simulink model "PedalCmd"  (R2016a)
settings: Solver=FixedStepDiscrete  StartTime=0.0  StopTime=2  FixedStep=0.1  RelTol=1e-3
PostLoadFcn:
  | CruiseControl_dd;
undefined symbols (not defined in the file): PedalCmdY, SpeedDelX
settings Model: Creator=The MathWorks Inc.  LastModifiedBy=colosky
settings DataIOCC: LimitDataPoints=on  SaveFormat=Array  SaveOutput=off  SaveTime=off
settings OptimizationCC: ConditionallyExecuteInputs=off  DefaultParameterBehavior=Inlined  InlineInvariantSignals=on  ExpressionDepthLimit=2147483647  InitFltsAndDblsToZero=on  NoFixptDivByZeroProtection=on  OptimizeModelRefInitCode=on
settings DebuggingCC: SaveWithParameterizedLinksMsg=none  UnderspecifiedInitializationDetection=Classic  MergeDetectMultiDrivingBlocksExec=none  SolverPrmCheckMsg=warning  FcnCallInpInsideContextMsg=UseLocalSettings  AllowSymbolicDim=off  StateNameClashWarn=warning  StrictBusMsg=ErrorOnBusTreatedAsVector
settings HardwareCC: ProdBitPerPointer=32  ProdLargestAtomicFloat=None  ProdIntDivRoundTo=Undefined  ProdEndianess=Unspecified  ProdWordSize=32  ProdHWDeviceType=32-bit Generic
settings ModelReferenceCC: ModelReferenceNumInstancesAllowed=Single  PropagateSignalLabelsOutOfModel=off
settings SFSimCC: SimParseCustomCode=off
settings RTWCC: SystemTargetFile=ert.tlc  TemplateMakefile=ert_default_tmf  GenerateReport=on  IncludeHyperlinkInReport=on  LaunchReport=on  PortableWordSizes=on  GenerateTraceInfo=on  GenerateTraceReport=on  GenerateTraceReportSl=on  GenerateTraceReportSf=on  GenerateTraceReportEml=on
settings CodeAppCC: IgnoreCustomStorageClasses=off  CustomSymbolStrGlobalVar=$N$M
settings ERTTargetCC: GenerateSampleERTMain=on  InlinedParameterPlacement=NonHierarchical  ERTCustomFileTemplate=example_file_process.tlc  ConvertIfToSwitch=off  SuppressUnreachableDefaultCases=off
settings ConfigComp: CovEnable=on  CovScope=ReferencedModels  CovIncludeTopModel=off  RecordCoverage=on  CovMetricSettings=dcme  CovHtmlReporting=off  CovSaveCumulativeToWorkspaceVar=off  CovSaveSingleToWorkspaceVar=off  CovModelRefEnable=Off  CovSFcnEnable=off  DVMode=DesignErrorDetection  DVMaxProcessTime=3000  DVDisplayUnsatisfiableObjectives=on  DVAutomaticStubbing=off  DVMakeOutputFilesUnique=off  DVMaxTestCaseSteps=500  DVTestSuiteOptimization=CombinedObjectives (Nonlinear Extended)  DVAssertions=EnableAll  DVProofAssumptions=EnableAll  DVCoverageDataFile=cumcov_PartCvg.cvt  DVIncludeRelationalBoundary=on  DVDetectIntegerOverflow=off  DVDetectDeadLogic=on  DVDetectActiveLogic=on  DVMaxViolationSteps=50  DVSaveExpectedOutput=on  DVSaveHarnessModel=on  DVHarnessModelFileName=$ModelName$_harness_SLDV  DVModelReferenceHarness=on  DVReportIncludeGraphics=on  PSVerificationMode=BugFinder  PSOpenProjectManager=on  PSParamRangeMode=DesignMinMax  PSAutoStubLUT=off

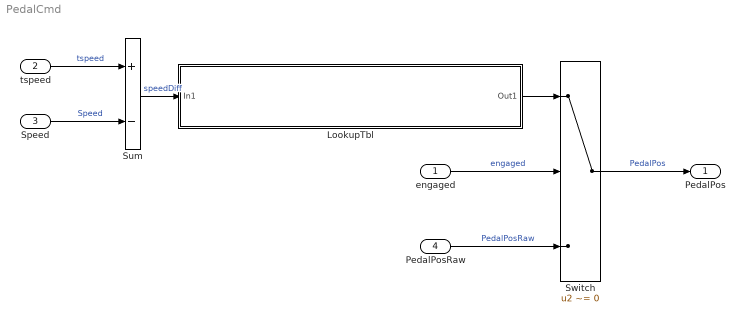
== system PedalCmd ==
  engaged : Inport  OutDataTypeStr=boolean  PortDimensions=1
  tspeed : Inport  Port=2  OutDataTypeStr=uint8  PortDimensions=1
  Speed : Inport  Port=3  OutDataTypeStr=uint8  PortDimensions=1
  PedalPosRaw : Inport  Port=4  OutDataTypeStr=single  PortDimensions=1
  LookupTbl : Subsystem
  Sum : Sum  Inputs=+-  AccumDataTypeStr=int8  OutDataTypeStr=int8  InputSameDT=on
  Switch : Switch  Criteria=u2 ~= 0
  PedalPos : Outport
  wires:
  engaged/1 -> Switch/2  "engaged"
  PedalPosRaw/1 -> Switch/3  "PedalPosRaw"
  Switch/1 -> PedalPos/1  "PedalPos"
  Speed/1 -> Sum/2  "Speed"
  tspeed/1 -> Sum/1  "tspeed"
  Sum/1 -> LookupTbl/1(In1)  "speedDiff"
  LookupTbl/1(Out1) -> Switch/1

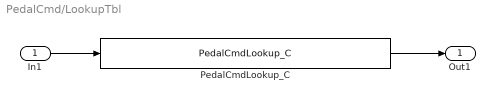
== system PedalCmd/LookupTbl ==
  In1 : Inport
  PedalCmdLookup_C : S-Function  FunctionName=PedalCmdLookup_C  Parameters=SParameter1, SParameter2  SFunctionDeploymentMode=off  EnableBusSupport=off  mask(Legacy Function){SFunctionSpec=single y1 = Lookup1D_C(int8 u1,int8 p1[],single p2[]), SParameter1=SpeedDelX, SParameter2=PedalCmdY, ShowSpec=on}
      mask prompts: SParameter1 "P1:"; SParameter2 "P2:"; ShowSpec "Display function specification"
      mask help:
      | This block allows you to call the legacy functions specified by the following Legacy Code Tool definition:
      | def.SFunctionName = 'PedalCmdLookup_C';
      | def.OutputFcnSpec = 'single y1 = Lookup1D_C(int8 u1,int8 p1[],single p2[])';
      | def.HeaderFiles = {'Lookup1D_C.h'};
      | def.SourceFiles = {'Lookup1D_C.c'};
      | def.Options.supportCoverageAndDesignVerifier = true;
      mask Help: <p>This block was generated automatically by the Legacy Code Tool. For detailed help on this tool, call<a href="matlab:legacy_code('help')"> legacy_code('help')</a>.</p>
      mask Callback ShowSpec:
      | if strcmp(get_param(gcbh, 'ShowSpec'), 'on')
      |   set_param(gcbh, 'MaskDisplay', sprintf('fprintf(''%s'');', get_param(gcbh, 'SFunctionSpec')));
      | else
      |   set_param(gcbh, 'MaskDisplay', sprintf('fprintf(''%s'');', get_param(gcbh, 'FunctionName')));
      | end
      mask Display: fprintf('single y1 = Lookup1D_C(int8 u1,int8 p1[],single p2[])');
  Out1 : Outport
  wires:
  In1/1 -> PedalCmdLookup_C/1
  PedalCmdLookup_C/1 -> Out1/1
